simulink subsystem "OffsetRemover"  (R2024b)
settings: Solver=VariableStepAuto  StartTime=0.0  StopTime=10.0  RelTol=1e-3
libraries: dspstat3 x1
settings Model: Creator=JesseJabezArendse  LastModifiedBy=JesseJabezArendse
settings RTWCC: GPUComputeCapability=3.5

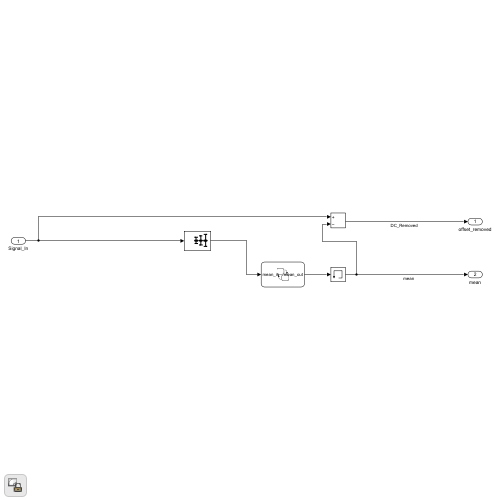
[thumbnail: Simulink's stored preview of the top-level diagram]
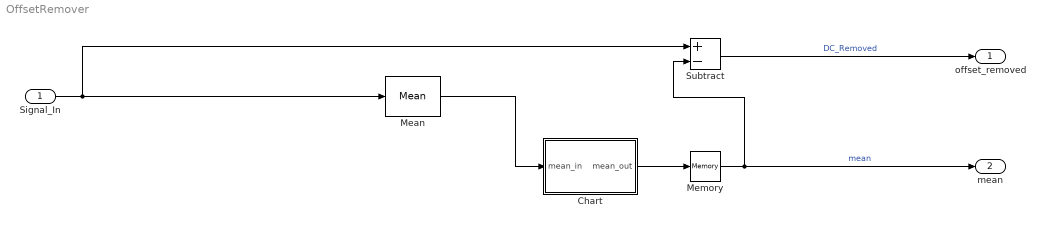
== system OffsetRemover ==
  Signal_In : Inport  OutDataTypeStr=single
  Chart : Stateflow chart  TreatAsAtomicUnit=on
  Mean : dspstat3/Mean  run=on  reset_popup=None  directionMode=Entire input  dimension=1  roiEnable=off  roiType=Rectangles  roiPortion=Entire ROI  roiOutput=Individual statistics for each ROI  roiFlag=off  roundingMode=Floor  overflowMode=off  outputMin=[]  outputMax=[]
  Memory : Memory
  Subtract : Sum  Inputs=+-  OutDataTypeStr=single
  offset_removed : Outport  OutDataTypeStr=single
  mean : Outport  Port=2  OutDataTypeStr=single
  wires:
  Signal_In/1 -> Subtract/1, Mean/1
  Memory/1 -> Subtract/2, mean/1  "mean"
  Subtract/1 -> offset_removed/1  "DC_Removed"
  Chart/1(mean_out) -> Memory/1
  Mean/1 -> Chart/1(mean_in)

== stateflow chart OffsetRemover/Chart ==
  state Wait
  state Done
    entry:
    mean_out = mean_in;
  (default) -> Wait
  Wait -> Done : after(0.2,sec)
  data: mean_out output single size=1 =0; mean_in input single size=1
